simulink subsystem "ReIm2MagAngle"  (R2023b)
settings: Solver=VariableStepAuto  StartTime=0.0  StopTime=10.0  RelTol=1e-3
settings Model: Creator=Veimar  LastModifiedBy=Veimar

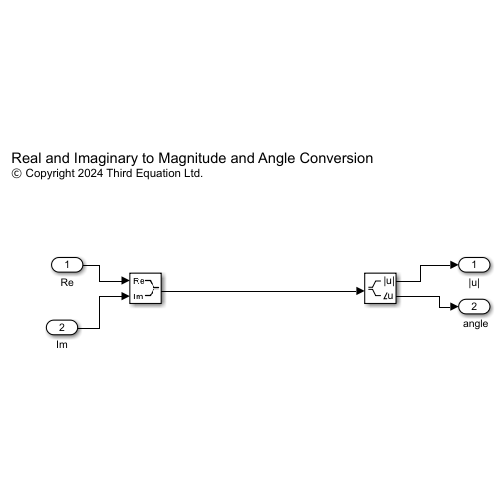
[thumbnail: Simulink's stored preview of the top-level diagram]
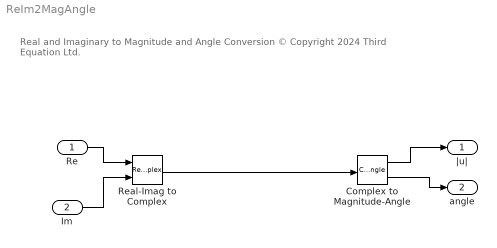
== system ReIm2MagAngle ==
  note: Real and Imaginary to Magnitude and Angle Conversion
      | © Copyright 2024 Third Equation Ltd.
  Re : Inport
  Im : Inport  Port=2
  Complex to Magnitude-Angle : ComplexToMagnitudeAngle
  Real-Imag to Complex : RealImagToComplex
  |u| : Outport
  " angle" : Outport  Port=2
  wires:
  Re/1 -> Real-Imag to Complex/1
  Complex to Magnitude-Angle/1 -> |u|/1
  Complex to Magnitude-Angle/2 -> " angle"/1
  Real-Imag to Complex/1 -> Complex to Magnitude-Angle/1
  Im/1 -> Real-Imag to Complex/2
